simulink model "Automatic_turn_light_feature_discrete_with_plant_model"  (R2026a)
settings: Solver=VariableStepAuto  StopTime=100
libraries: arduinolib x5, SignalEditorBlockLib x1
settings Model: SILPILSystemUnderTest=refmodels  Creator=irfan  LastModifiedBy=irfan

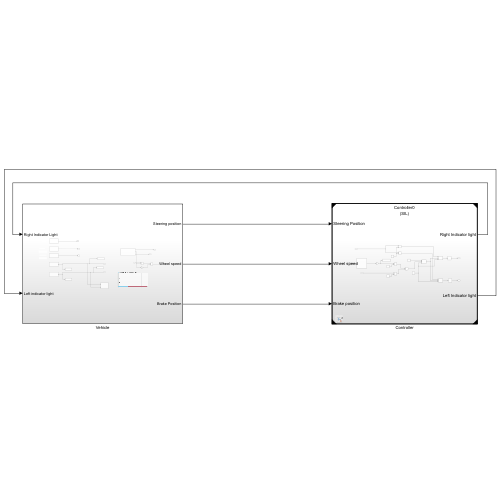
[thumbnail: Simulink's stored preview of the top-level diagram]
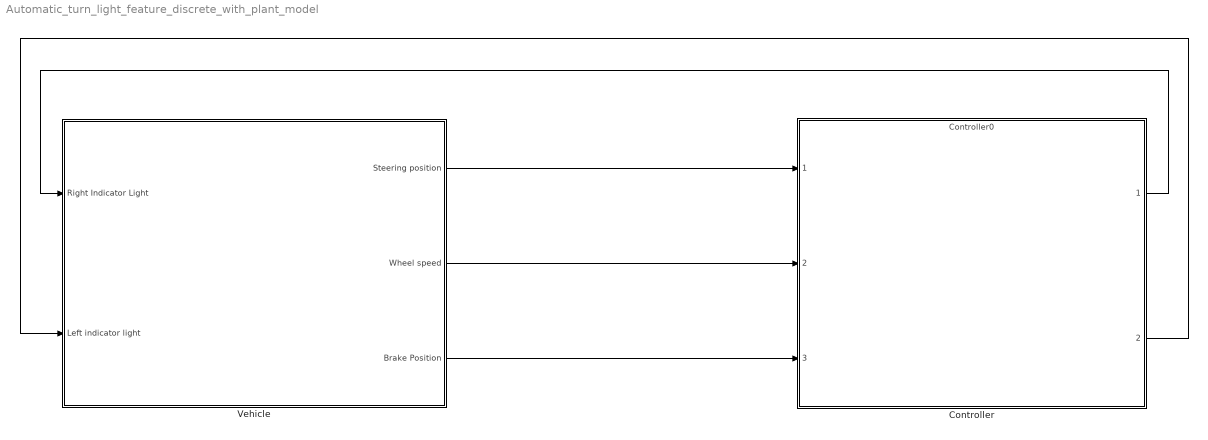
== system Automatic_turn_light_feature_discrete_with_plant_model ==
  Controller : ModelReference  ModelNameDialog=Controller0  SimulationMode=Software-in-the-loop (SIL)  ModelReferenceVersion=1.18
  Vehicle : Subsystem
  wires:
  Controller/1 -> Vehicle/1(Right Indicator Light)
  Controller/2 -> Vehicle/2(Left indicator light)
  Vehicle/1(Steering position) -> Controller/1
  Vehicle/2(Wheel speed) -> Controller/2
  Vehicle/3(Brake Position) -> Controller/3

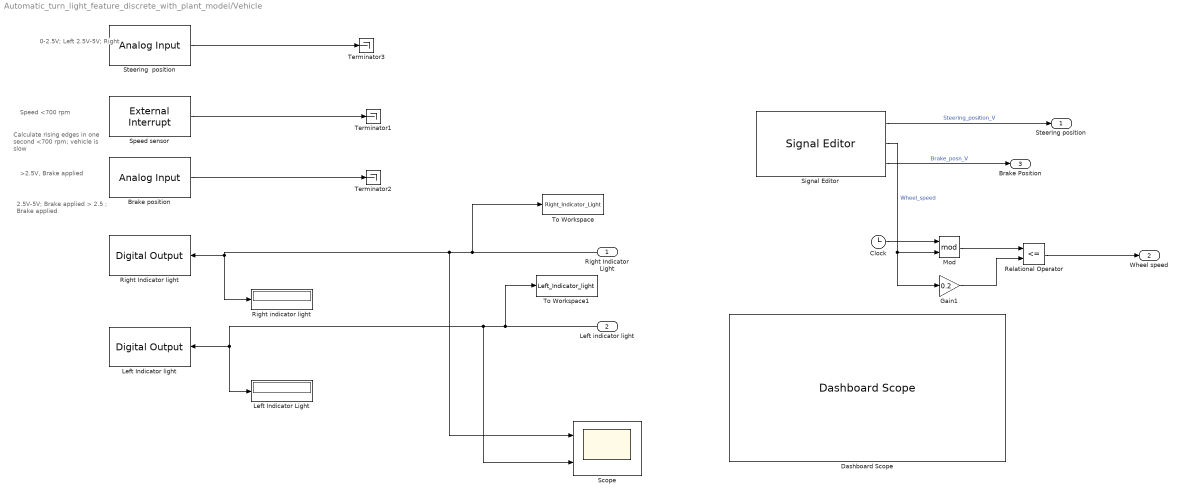
== system Automatic_turn_light_feature_discrete_with_plant_model/Vehicle ==
  note: Calculate rising edges
      | in one second
      | <700 rpm; vehicle is slow
  note: 2.5V-5V; Brake applied
      | > 2.5 ; Brake applied
  note: Speed <700 rpm
  note: >2.5V, Brake applied
  note: 0-2.5V; Left
      | 2.5V-5V; Right
  Right Indicator Light : Inport
  Left indicator light : Inport  Port=2
  Brake position : arduinolib/Analog Input  pinNumber=2  ReadResultsOnly=off  ConversionTriggerSource=Software  ExternalTriggerType=uint32( 0 )  OutputDataType=uint16  EnableConversionCompleteNotify=off  EnableOuputStatus=off  SampleTime=-1  blockPlatform=arduino
  Clock : Clock
  Dashboard Scope : DashboardScope  TicksPosition=Inside  FontColor=[0.0, 0.0, 0.0]
  Gain1 : Gain  Gain=0.2
  Left Indicator Light : Display
  Left Indicator light : arduinolib/Digital Output  pinNumber=12  Direction=output  blockPlatform=arduino
  Mod : Math  Operator=mod
  Relational Operator : RelationalOperator  Operator=<=  OutDataTypeStr=Inherit: Inherit via back propagation  RndMeth=Simplest  InputSameDT=off
  Right Indicator light : arduinolib/Digital Output  pinNumber=13  Direction=output  blockPlatform=arduino
  Right indicator light : Display
  Scope : Scope  NumInputPorts=2
      settings: ActiveDisplayYMinimum=-0.12499999999999997  ActiveDisplayYMaximum=1.125
  Signal Editor : SignalEditorBlockLib/Signal Editor  FileName=C:\Users\irfan\OneDrive\Documents\MATLAB\Blitz_Project\Signal_builder.mat  ActiveScenario=Test1  ActiveSignal=Steering_Position  IsBus=off  OutputBusObjectStr=Bus: BusObject  SampleTime=0  ZeroCross=off  OutputAfterFinalValue=Setting to zero  Unit=inherit  PreserveSignalName=on  ApplySigPropsToAllScenarios=on  ApplySigPropsToAllSignals=off  SignalPropertySource=Dialog parameters
  Speed sensor : arduinolib/External Interrupt  Pin=2  PullUp=off  Mode=RISING  InterruptSimulationInput=off
  Steering  position : arduinolib/Analog Input  pinNumber=1  ReadResultsOnly=off  ConversionTriggerSource=Software  ExternalTriggerType=uint32( 0 )  OutputDataType=uint16  EnableConversionCompleteNotify=off  EnableOuputStatus=off  SampleTime=-1  blockPlatform=arduino
  Terminator1 : Terminator
  Terminator2 : Terminator
  Terminator3 : Terminator
  To Workspace : ToWorkspace  VariableName=Right_Indicator_Light  SaveFormat=Timeseries  SampleTime=-1
  To Workspace1 : ToWorkspace  VariableName=Left_Indicator_light  SaveFormat=Timeseries  SampleTime=-1
  Steering position : Outport
  Wheel speed : Outport  Port=2
  Brake Position : Outport  Port=3
  wires:
  Left indicator light/1 -> To Workspace1/1, Scope/2, Left Indicator Light/1, Left Indicator light/1
  Right Indicator Light/1 -> To Workspace/1, Scope/1, Right indicator light/1, Right Indicator light/1
  Signal Editor/2 -> Gain1/1, Mod/2  "Wheel_speed"
  Signal Editor/1 -> Steering position/1  "Steering_position_V"
  Signal Editor/3 -> Brake Position/1  "Brake_posn_V"
  Speed sensor/1 -> Terminator1/1
  Brake position/1 -> Terminator2/1
  Clock/1 -> Mod/1
  Mod/1 -> Relational Operator/1
  Gain1/1 -> Relational Operator/2
  Relational Operator/1 -> Wheel speed/1
  Steering  position/1 -> Terminator3/1
